simulink model "model"  (R2014a)
settings: Solver=VariableStepAuto  StartTime=0.0  StopTime=10.0  RelTol=1e-3
libraries: powerlib x113
settings Model: Creator=lej  LastModifiedBy=leimhofe
settings DataIOCC: SaveFormat=Dataset
settings OptimizationCC: SimCompilerOptimization=off
settings DebuggingCC: MergeDetectMultiDrivingBlocksExec=error  SolverPrmCheckMsg=none  FrameProcessingCompatibilityMsg=error  AllowSymbolicDim=off
settings HardwareCC: ProdBitPerPointer=64  ProdLargestAtomicFloat=Float  ProdIntDivRoundTo=Zero  ProdEndianess=LittleEndian  ProdWordSize=64  ProdHWDeviceType=Intel->x86-64 (Windows64)
settings RTWCC: RTWCompilerOptimization=off
settings GRTTargetCC: GeneratePreprocessorConditionals=Use local settings
settings ConfigComp: CovMetricSettings=dw  CovHtmlReporting=on  CovSaveCumulativeToWorkspaceVar=on  CovSaveSingleToWorkspaceVar=on  CovExternalEMLEnable=off

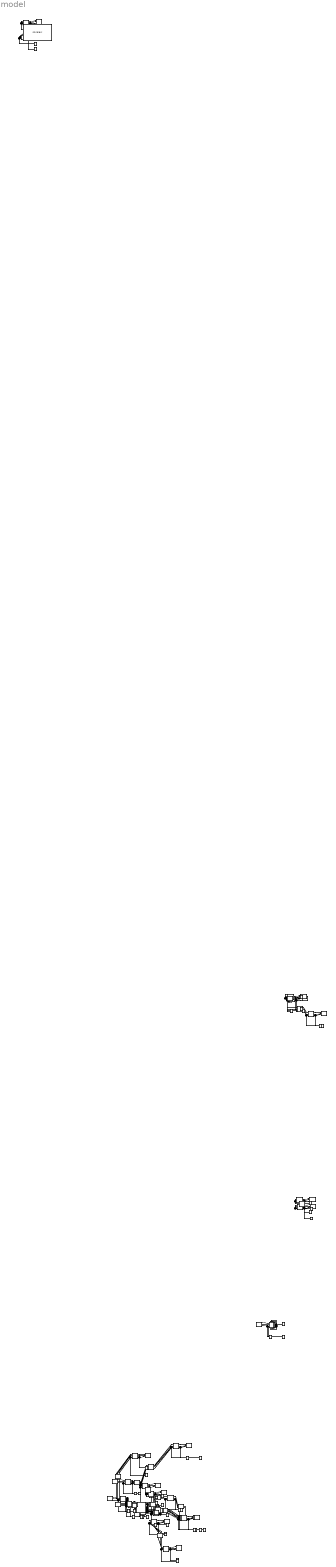
== system model ==
  note: 110000 Volts Power Line
  note: 220000 Volts Power Line
  note: 500000 Volts Power Line
  G_308292616_ : powerlib/Electrical Sources/Three-Phase Source  Voltage=220000  PhaseAngle=0  Frequency=60  InternalConnection=Yg  SpecifyImpedance=on  Resistance=0.8929  Inductance=16.58e-3  ShortCircuitLevel=100e6  BaseVoltage=220000  XRratio=7  BusType=swing  Pref=0  Qref=0  Qmin=-inf  Qmax=inf
  G_400202736_ : powerlib/Electrical Sources/Three-Phase Source  Voltage=220000  PhaseAngle=0  Frequency=60  InternalConnection=Yg  SpecifyImpedance=on  Resistance=0.8929  Inductance=16.58e-3  ShortCircuitLevel=100e6  BaseVoltage=220000  XRratio=7  BusType=swing  Pref=0  Qref=0  Qmin=-inf  Qmax=inf
  L_{251790836,251794098,277519190,306259034..306259035,306295540,306440155,308292630,315766015,318268202,400413519,400413521} (12 alike) : powerlib/Elements/Three-Phase Series RLC Load  LConnTagsString=A|B|C  Configuration=Y (grounded)  NominalVoltage=220000  NominalFrequency=60  ActivePower=100000  InductivePower=100  CapacitivePower=100  Measurements=None  LoadType=constant Z
  L_{272740093,306440153,315553115,401274166,401334056,401447890} (6 alike) : powerlib/Elements/Three-Phase Series RLC Load  LConnTagsString=A|B|C  Configuration=Y (grounded)  NominalVoltage=500000  NominalFrequency=60  ActivePower=100000  InductivePower=100  CapacitivePower=100  Measurements=None  LoadType=constant Z
  L_{306295536,307638314,317106134..317106135} (4 alike) : powerlib/Elements/Three-Phase Series RLC Load  LConnTagsString=A|B|C  Configuration=Y (grounded)  NominalVoltage=110000  NominalFrequency=60  ActivePower=100000  InductivePower=100  CapacitivePower=100  Measurements=None  LoadType=constant Z
  T_251790836__ : powerlib/Elements/Three-Phase Transformer (Two Windings)  Winding1Connection=Yg  UNITS=pu  NominalPower=[ 250e6 , 60 ]  Winding1=[220000,0.002,0.08]  Winding2Connection=Yg  Winding2=[220000,0.002,0.08]  SetSaturation=off  Rm=500  Lm=500  Saturation=[ 0,0 ; 0.0024,1.2 ; 1.0,1.52 ]  Hysteresis=off  DataFile='hysteresis'  SetInitialFlux=off  InitialFluxes=[ 0.8 , -0.8 , 0.7 ]  Measurements=None  MoreParameters=off  BreakLoop=off  DataType=off  TransfoNumber=1
  T_251794098__ : powerlib/Elements/Three-Phase Transformer (Two Windings)  Winding1Connection=Yg  UNITS=pu  NominalPower=[ 250e6 , 60 ]  Winding1=[220000,0.002,0.08]  Winding2Connection=Yg  Winding2=[220000,0.002,0.08]  SetSaturation=off  Rm=500  Lm=500  Saturation=[ 0,0 ; 0.0024,1.2 ; 1.0,1.52 ]  Hysteresis=off  DataFile='hysteresis'  SetInitialFlux=off  InitialFluxes=[ 0.8 , -0.8 , 0.7 ]  Measurements=None  MoreParameters=off  BreakLoop=off  DataType=off  TransfoNumber=1
  T_272740093_500000_Trạm_500KV_Phú_Mỹ : powerlib/Elements/Three-Phase Transformer (Two Windings)  Winding1Connection=Yg  UNITS=pu  NominalPower=[ 250e6 , 60 ]  Winding1=[500000,0.002,0.08]  Winding2Connection=Yg  Winding2=[500000,0.002,0.08]  SetSaturation=off  Rm=500  Lm=500  Saturation=[ 0,0 ; 0.0024,1.2 ; 1.0,1.52 ]  Hysteresis=off  DataFile='hysteresis'  SetInitialFlux=off  InitialFluxes=[ 0.8 , -0.8 , 0.7 ]  Measurements=None  MoreParameters=off  BreakLoop=off  DataType=off  TransfoNumber=1
  T_277519190__ : powerlib/Elements/Three-Phase Transformer (Two Windings)  Winding1Connection=Yg  UNITS=pu  NominalPower=[ 250e6 , 60 ]  Winding1=[220000,0.002,0.08]  Winding2Connection=Yg  Winding2=[220000,0.002,0.08]  SetSaturation=off  Rm=500  Lm=500  Saturation=[ 0,0 ; 0.0024,1.2 ; 1.0,1.52 ]  Hysteresis=off  DataFile='hysteresis'  SetInitialFlux=off  InitialFluxes=[ 0.8 , -0.8 , 0.7 ]  Measurements=None  MoreParameters=off  BreakLoop=off  DataType=off  TransfoNumber=1
  T_306259034__ : powerlib/Elements/Three-Phase Transformer (Two Windings)  Winding1Connection=Yg  UNITS=pu  NominalPower=[ 250e6 , 60 ]  Winding1=[220000,0.002,0.08]  Winding2Connection=Yg  Winding2=[220000,0.002,0.08]  SetSaturation=off  Rm=500  Lm=500  Saturation=[ 0,0 ; 0.0024,1.2 ; 1.0,1.52 ]  Hysteresis=off  DataFile='hysteresis'  SetInitialFlux=off  InitialFluxes=[ 0.8 , -0.8 , 0.7 ]  Measurements=None  MoreParameters=off  BreakLoop=off  DataType=off  TransfoNumber=1
  T_306259035__ : powerlib/Elements/Three-Phase Transformer (Two Windings)  Winding1Connection=Yg  UNITS=pu  NominalPower=[ 250e6 , 60 ]  Winding1=[220000,0.002,0.08]  Winding2Connection=Yg  Winding2=[220000,0.002,0.08]  SetSaturation=off  Rm=500  Lm=500  Saturation=[ 0,0 ; 0.0024,1.2 ; 1.0,1.52 ]  Hysteresis=off  DataFile='hysteresis'  SetInitialFlux=off  InitialFluxes=[ 0.8 , -0.8 , 0.7 ]  Measurements=None  MoreParameters=off  BreakLoop=off  DataType=off  TransfoNumber=1
  T_306295536_500000_Trạm_500KV_Nhà_Bè : powerlib/Elements/Three-Phase Transformer (Three Windings)  Winding1Connection=Yg  UNITS=pu  NominalPower=[ 250e6 , 60 ]  Winding1=[500000,0.002,0.08]  Winding2Connection=Yg  Winding2=[220000,0.002,0.08]  Winding3Connection=Yg  Winding3=[110000,0.002,0.08]  SetSaturation=off  Rm=500  Lm=500  Saturation=[ 0,0 ; 0.0024,1.2 ; 1.0,1.52 ]  Hysteresis=off  DataFile='hysteresis'  SetInitialFlux=off  InitialFluxes=[0.8 -0.8 0.7]  Measurements=None  MoreParameters=off  BreakLoop=off  DataType=off  TransfoNumber=1
  T_306295540__ : powerlib/Elements/Three-Phase Transformer (Two Windings)  Winding1Connection=Yg  UNITS=pu  NominalPower=[ 250e6 , 60 ]  Winding1=[220000,0.002,0.08]  Winding2Connection=Yg  Winding2=[220000,0.002,0.08]  SetSaturation=off  Rm=500  Lm=500  Saturation=[ 0,0 ; 0.0024,1.2 ; 1.0,1.52 ]  Hysteresis=off  DataFile='hysteresis'  SetInitialFlux=off  InitialFluxes=[ 0.8 , -0.8 , 0.7 ]  Measurements=None  MoreParameters=off  BreakLoop=off  DataType=off  TransfoNumber=1
  T_306440153__ : powerlib/Elements/Three-Phase Transformer (Two Windings)  Winding1Connection=Yg  UNITS=pu  NominalPower=[ 250e6 , 60 ]  Winding1=[500000,0.002,0.08]  Winding2Connection=Yg  Winding2=[500000,0.002,0.08]  SetSaturation=off  Rm=500  Lm=500  Saturation=[ 0,0 ; 0.0024,1.2 ; 1.0,1.52 ]  Hysteresis=off  DataFile='hysteresis'  SetInitialFlux=off  InitialFluxes=[ 0.8 , -0.8 , 0.7 ]  Measurements=None  MoreParameters=off  BreakLoop=off  DataType=off  TransfoNumber=1
  T_306440155__ : powerlib/Elements/Three-Phase Transformer (Two Windings)  Winding1Connection=Yg  UNITS=pu  NominalPower=[ 250e6 , 60 ]  Winding1=[220000,0.002,0.08]  Winding2Connection=Yg  Winding2=[220000,0.002,0.08]  SetSaturation=off  Rm=500  Lm=500  Saturation=[ 0,0 ; 0.0024,1.2 ; 1.0,1.52 ]  Hysteresis=off  DataFile='hysteresis'  SetInitialFlux=off  InitialFluxes=[ 0.8 , -0.8 , 0.7 ]  Measurements=None  MoreParameters=off  BreakLoop=off  DataType=off  TransfoNumber=1
  T_307638314__ : powerlib/Elements/Three-Phase Transformer (Two Windings)  Winding1Connection=Yg  UNITS=pu  NominalPower=[ 250e6 , 60 ]  Winding1=[220000,0.002,0.08]  Winding2Connection=Yg  Winding2=[110000,0.002,0.08]  SetSaturation=off  Rm=500  Lm=500  Saturation=[ 0,0 ; 0.0024,1.2 ; 1.0,1.52 ]  Hysteresis=off  DataFile='hysteresis'  SetInitialFlux=off  InitialFluxes=[ 0.8 , -0.8 , 0.7 ]  Measurements=None  MoreParameters=off  BreakLoop=off  DataType=off  TransfoNumber=1
  T_308292630__ : powerlib/Elements/Three-Phase Transformer (Two Windings)  Winding1Connection=Yg  UNITS=pu  NominalPower=[ 250e6 , 60 ]  Winding1=[220000,0.002,0.08]  Winding2Connection=Yg  Winding2=[220000,0.002,0.08]  SetSaturation=off  Rm=500  Lm=500  Saturation=[ 0,0 ; 0.0024,1.2 ; 1.0,1.52 ]  Hysteresis=off  DataFile='hysteresis'  SetInitialFlux=off  InitialFluxes=[ 0.8 , -0.8 , 0.7 ]  Measurements=None  MoreParameters=off  BreakLoop=off  DataType=off  TransfoNumber=1
  T_315553115__Phú_Lâm : powerlib/Elements/Three-Phase Transformer (Two Windings)  Winding1Connection=Yg  UNITS=pu  NominalPower=[ 250e6 , 60 ]  Winding1=[500000,0.002,0.08]  Winding2Connection=Yg  Winding2=[500000,0.002,0.08]  SetSaturation=off  Rm=500  Lm=500  Saturation=[ 0,0 ; 0.0024,1.2 ; 1.0,1.52 ]  Hysteresis=off  DataFile='hysteresis'  SetInitialFlux=off  InitialFluxes=[ 0.8 , -0.8 , 0.7 ]  Measurements=None  MoreParameters=off  BreakLoop=off  DataType=off  TransfoNumber=1
  T_315766015__ : powerlib/Elements/Three-Phase Transformer (Two Windings)  Winding1Connection=Yg  UNITS=pu  NominalPower=[ 250e6 , 60 ]  Winding1=[220000,0.002,0.08]  Winding2Connection=Yg  Winding2=[220000,0.002,0.08]  SetSaturation=off  Rm=500  Lm=500  Saturation=[ 0,0 ; 0.0024,1.2 ; 1.0,1.52 ]  Hysteresis=off  DataFile='hysteresis'  SetInitialFlux=off  InitialFluxes=[ 0.8 , -0.8 , 0.7 ]  Measurements=None  MoreParameters=off  BreakLoop=off  DataType=off  TransfoNumber=1
  T_317106134__ : powerlib/Elements/Three-Phase Transformer (Two Windings)  Winding1Connection=Yg  UNITS=pu  NominalPower=[ 250e6 , 60 ]  Winding1=[110000,0.002,0.08]  Winding2Connection=Yg  Winding2=[110000,0.002,0.08]  SetSaturation=off  Rm=500  Lm=500  Saturation=[ 0,0 ; 0.0024,1.2 ; 1.0,1.52 ]  Hysteresis=off  DataFile='hysteresis'  SetInitialFlux=off  InitialFluxes=[ 0.8 , -0.8 , 0.7 ]  Measurements=None  MoreParameters=off  BreakLoop=off  DataType=off  TransfoNumber=1
  T_317106135__ : powerlib/Elements/Three-Phase Transformer (Two Windings)  Winding1Connection=Yg  UNITS=pu  NominalPower=[ 250e6 , 60 ]  Winding1=[110000,0.002,0.08]  Winding2Connection=Yg  Winding2=[110000,0.002,0.08]  SetSaturation=off  Rm=500  Lm=500  Saturation=[ 0,0 ; 0.0024,1.2 ; 1.0,1.52 ]  Hysteresis=off  DataFile='hysteresis'  SetInitialFlux=off  InitialFluxes=[ 0.8 , -0.8 , 0.7 ]  Measurements=None  MoreParameters=off  BreakLoop=off  DataType=off  TransfoNumber=1
  T_318268202__ : powerlib/Elements/Three-Phase Transformer (Two Windings)  Winding1Connection=Yg  UNITS=pu  NominalPower=[ 250e6 , 60 ]  Winding1=[220000,0.002,0.08]  Winding2Connection=Yg  Winding2=[220000,0.002,0.08]  SetSaturation=off  Rm=500  Lm=500  Saturation=[ 0,0 ; 0.0024,1.2 ; 1.0,1.52 ]  Hysteresis=off  DataFile='hysteresis'  SetInitialFlux=off  InitialFluxes=[ 0.8 , -0.8 , 0.7 ]  Measurements=None  MoreParameters=off  BreakLoop=off  DataType=off  TransfoNumber=1
  T_400413519__ : powerlib/Elements/Three-Phase Transformer (Two Windings)  Winding1Connection=Yg  UNITS=pu  NominalPower=[ 250e6 , 60 ]  Winding1=[220000,0.002,0.08]  Winding2Connection=Yg  Winding2=[220000,0.002,0.08]  SetSaturation=off  Rm=500  Lm=500  Saturation=[ 0,0 ; 0.0024,1.2 ; 1.0,1.52 ]  Hysteresis=off  DataFile='hysteresis'  SetInitialFlux=off  InitialFluxes=[ 0.8 , -0.8 , 0.7 ]  Measurements=None  MoreParameters=off  BreakLoop=off  DataType=off  TransfoNumber=1
  T_400413521__ : powerlib/Elements/Three-Phase Transformer (Two Windings)  Winding1Connection=Yg  UNITS=pu  NominalPower=[ 250e6 , 60 ]  Winding1=[220000,0.002,0.08]  Winding2Connection=Yg  Winding2=[220000,0.002,0.08]  SetSaturation=off  Rm=500  Lm=500  Saturation=[ 0,0 ; 0.0024,1.2 ; 1.0,1.52 ]  Hysteresis=off  DataFile='hysteresis'  SetInitialFlux=off  InitialFluxes=[ 0.8 , -0.8 , 0.7 ]  Measurements=None  MoreParameters=off  BreakLoop=off  DataType=off  TransfoNumber=1
  T_401274166__ : powerlib/Elements/Three-Phase Transformer (Two Windings)  Winding1Connection=Yg  UNITS=pu  NominalPower=[ 250e6 , 60 ]  Winding1=[500000,0.002,0.08]  Winding2Connection=Yg  Winding2=[500000,0.002,0.08]  SetSaturation=off  Rm=500  Lm=500  Saturation=[ 0,0 ; 0.0024,1.2 ; 1.0,1.52 ]  Hysteresis=off  DataFile='hysteresis'  SetInitialFlux=off  InitialFluxes=[ 0.8 , -0.8 , 0.7 ]  Measurements=None  MoreParameters=off  BreakLoop=off  DataType=off  TransfoNumber=1
  T_401334056__ : powerlib/Elements/Three-Phase Transformer (Two Windings)  Winding1Connection=Yg  UNITS=pu  NominalPower=[ 250e6 , 60 ]  Winding1=[500000,0.002,0.08]  Winding2Connection=Yg  Winding2=[500000,0.002,0.08]  SetSaturation=off  Rm=500  Lm=500  Saturation=[ 0,0 ; 0.0024,1.2 ; 1.0,1.52 ]  Hysteresis=off  DataFile='hysteresis'  SetInitialFlux=off  InitialFluxes=[ 0.8 , -0.8 , 0.7 ]  Measurements=None  MoreParameters=off  BreakLoop=off  DataType=off  TransfoNumber=1
  T_401447890__ : powerlib/Elements/Three-Phase Transformer (Two Windings)  Winding1Connection=Yg  UNITS=pu  NominalPower=[ 250e6 , 60 ]  Winding1=[500000,0.002,0.08]  Winding2Connection=Yg  Winding2=[500000,0.002,0.08]  SetSaturation=off  Rm=500  Lm=500  Saturation=[ 0,0 ; 0.0024,1.2 ; 1.0,1.52 ]  Hysteresis=off  DataFile='hysteresis'  SetInitialFlux=off  InitialFluxes=[ 0.8 , -0.8 , 0.7 ]  Measurements=None  MoreParameters=off  BreakLoop=off  DataType=off  TransfoNumber=1
  _CN_251794098_220000_CN_251790836_220000 : powerlib/Elements/Distributed Parameters Line  Phases=3  Frequency=60  Resistance=[0.01273 0.3864]  Inductance="[0.9337e-3  4.1264e-3]"  Capacitance=[12.74e-9 7.751e-9]  Length=16.0988  x1=[0 0 0 0; 0.0001244 0 0 0; 0.0002488 0 0 0; 0.0003733 0 0 0; 0.0004977 0 0 0; 0.0006221 0 0 0]  x2=[0 0 0 0; 0.0001244 0 0 0; 0.0002488 0 0 0; 0.0003733 0 0 0; 0.0004977 0 0 0; 0.0006221 0 0 0]  x3=[0 0 0 0; 0.0001244 0 0 0; 0.0002488 0 0 0; 0.0003733 0 0 0; 0.0004977 0 0 0; 0.0006221 0 0 0]  x4=[0 0 0 0; 0.0001244 0 0 0; 0.0002488 0 0 0; 0.0003733 0 0 0; 0.0004977 0 0 0; 0.0006221 0 0 0]  x5=0  V1=ones(3,3)  V2=ones(3,3)  I1=ones(3,3)  I2=ones(3,3)  nHarmo=1  Measurements=None
  _CN_277519190_220000_CN_315766015_220000 : powerlib/Elements/Distributed Parameters Line  Phases=3  Frequency=60  Resistance=[0.01273 0.3864]  Inductance="[0.9337e-3  4.1264e-3]"  Capacitance=[12.74e-9 7.751e-9]  Length=24.7895  x1=[0 0 0 0; 0.0001244 0 0 0; 0.0002488 0 0 0; 0.0003733 0 0 0; 0.0004977 0 0 0; 0.0006221 0 0 0]  x2=[0 0 0 0; 0.0001244 0 0 0; 0.0002488 0 0 0; 0.0003733 0 0 0; 0.0004977 0 0 0; 0.0006221 0 0 0]  x3=[0 0 0 0; 0.0001244 0 0 0; 0.0002488 0 0 0; 0.0003733 0 0 0; 0.0004977 0 0 0; 0.0006221 0 0 0]  x4=[0 0 0 0; 0.0001244 0 0 0; 0.0002488 0 0 0; 0.0003733 0 0 0; 0.0004977 0 0 0; 0.0006221 0 0 0]  x5=0  V1=ones(3,3)  V2=ones(3,3)  I1=ones(3,3)  I2=ones(3,3)  nHarmo=1  Measurements=None
  _CN_306259035_220000_CN_306259034_220000 : powerlib/Elements/Distributed Parameters Line  Phases=3  Frequency=60  Resistance=[0.01273 0.3864]  Inductance="[0.9337e-3  4.1264e-3]"  Capacitance=[12.74e-9 7.751e-9]  Length=8.7616  x1=[0 0 0 0; 0.0001244 0 0 0; 0.0002488 0 0 0; 0.0003733 0 0 0; 0.0004977 0 0 0; 0.0006221 0 0 0]  x2=[0 0 0 0; 0.0001244 0 0 0; 0.0002488 0 0 0; 0.0003733 0 0 0; 0.0004977 0 0 0; 0.0006221 0 0 0]  x3=[0 0 0 0; 0.0001244 0 0 0; 0.0002488 0 0 0; 0.0003733 0 0 0; 0.0004977 0 0 0; 0.0006221 0 0 0]  x4=[0 0 0 0; 0.0001244 0 0 0; 0.0002488 0 0 0; 0.0003733 0 0 0; 0.0004977 0 0 0; 0.0006221 0 0 0]  x5=0  V1=ones(3,3)  V2=ones(3,3)  I1=ones(3,3)  I2=ones(3,3)  nHarmo=1  Measurements=None
  _CN_306259035_220000_CN_306440155_220000 : powerlib/Elements/Distributed Parameters Line  Phases=3  Frequency=60  Resistance=[0.01273 0.3864]  Inductance="[0.9337e-3  4.1264e-3]"  Capacitance=[12.74e-9 7.751e-9]  Length=62.0615  x1=[0 0 0 0; 0.0001244 0 0 0; 0.0002488 0 0 0; 0.0003733 0 0 0; 0.0004977 0 0 0; 0.0006221 0 0 0]  x2=[0 0 0 0; 0.0001244 0 0 0; 0.0002488 0 0 0; 0.0003733 0 0 0; 0.0004977 0 0 0; 0.0006221 0 0 0]  x3=[0 0 0 0; 0.0001244 0 0 0; 0.0002488 0 0 0; 0.0003733 0 0 0; 0.0004977 0 0 0; 0.0006221 0 0 0]  x4=[0 0 0 0; 0.0001244 0 0 0; 0.0002488 0 0 0; 0.0003733 0 0 0; 0.0004977 0 0 0; 0.0006221 0 0 0]  x5=0  V1=ones(3,3)  V2=ones(3,3)  I1=ones(3,3)  I2=ones(3,3)  nHarmo=1  Measurements=None
  _CN_306259035_220000_CN_318268202_220000 : powerlib/Elements/Distributed Parameters Line  Phases=3  Frequency=60  Resistance=[0.01273 0.3864]  Inductance="[0.9337e-3  4.1264e-3]"  Capacitance=[12.74e-9 7.751e-9]  Length=14.6107  x1=[0 0 0 0; 0.0001244 0 0 0; 0.0002488 0 0 0; 0.0003733 0 0 0; 0.0004977 0 0 0; 0.0006221 0 0 0]  x2=[0 0 0 0; 0.0001244 0 0 0; 0.0002488 0 0 0; 0.0003733 0 0 0; 0.0004977 0 0 0; 0.0006221 0 0 0]  x3=[0 0 0 0; 0.0001244 0 0 0; 0.0002488 0 0 0; 0.0003733 0 0 0; 0.0004977 0 0 0; 0.0006221 0 0 0]  x4=[0 0 0 0; 0.0001244 0 0 0; 0.0002488 0 0 0; 0.0003733 0 0 0; 0.0004977 0 0 0; 0.0006221 0 0 0]  x5=0  V1=ones(3,3)  V2=ones(3,3)  I1=ones(3,3)  I2=ones(3,3)  nHarmo=1  Measurements=None
  _CN_306295536_500000_CN_272740093_500000 : powerlib/Elements/Distributed Parameters Line  Phases=3  Frequency=60  Resistance=[0.01273 0.3864]  Inductance="[0.9337e-3  4.1264e-3]"  Capacitance=[12.74e-9 7.751e-9]  Length=42.5301  x1=[0 0 0 0; 0.0001244 0 0 0; 0.0002488 0 0 0; 0.0003733 0 0 0; 0.0004977 0 0 0; 0.0006221 0 0 0]  x2=[0 0 0 0; 0.0001244 0 0 0; 0.0002488 0 0 0; 0.0003733 0 0 0; 0.0004977 0 0 0; 0.0006221 0 0 0]  x3=[0 0 0 0; 0.0001244 0 0 0; 0.0002488 0 0 0; 0.0003733 0 0 0; 0.0004977 0 0 0; 0.0006221 0 0 0]  x4=[0 0 0 0; 0.0001244 0 0 0; 0.0002488 0 0 0; 0.0003733 0 0 0; 0.0004977 0 0 0; 0.0006221 0 0 0]  x5=0  V1=ones(3,3)  V2=ones(3,3)  I1=ones(3,3)  I2=ones(3,3)  nHarmo=1  Measurements=None
  _CN_306295536_500000_CN_315553115_500000 : powerlib/Elements/Distributed Parameters Line  Phases=3  Frequency=60  Resistance=[0.01273 0.3864]  Inductance="[0.9337e-3  4.1264e-3]"  Capacitance=[12.74e-9 7.751e-9]  Length=16.513  x1=[0 0 0 0; 0.0001244 0 0 0; 0.0002488 0 0 0; 0.0003733 0 0 0; 0.0004977 0 0 0; 0.0006221 0 0 0]  x2=[0 0 0 0; 0.0001244 0 0 0; 0.0002488 0 0 0; 0.0003733 0 0 0; 0.0004977 0 0 0; 0.0006221 0 0 0]  x3=[0 0 0 0; 0.0001244 0 0 0; 0.0002488 0 0 0; 0.0003733 0 0 0; 0.0004977 0 0 0; 0.0006221 0 0 0]  x4=[0 0 0 0; 0.0001244 0 0 0; 0.0002488 0 0 0; 0.0003733 0 0 0; 0.0004977 0 0 0; 0.0006221 0 0 0]  x5=0  V1=ones(3,3)  V2=ones(3,3)  I1=ones(3,3)  I2=ones(3,3)  nHarmo=1  Measurements=None
  _CN_306295540_220000_CN_277519190_220000 : powerlib/Elements/Distributed Parameters Line  Phases=3  Frequency=60  Resistance=[0.01273 0.3864]  Inductance="[0.9337e-3  4.1264e-3]"  Capacitance=[12.74e-9 7.751e-9]  Length=37.7221  x1=[0 0 0 0; 0.0001244 0 0 0; 0.0002488 0 0 0; 0.0003733 0 0 0; 0.0004977 0 0 0; 0.0006221 0 0 0]  x2=[0 0 0 0; 0.0001244 0 0 0; 0.0002488 0 0 0; 0.0003733 0 0 0; 0.0004977 0 0 0; 0.0006221 0 0 0]  x3=[0 0 0 0; 0.0001244 0 0 0; 0.0002488 0 0 0; 0.0003733 0 0 0; 0.0004977 0 0 0; 0.0006221 0 0 0]  x4=[0 0 0 0; 0.0001244 0 0 0; 0.0002488 0 0 0; 0.0003733 0 0 0; 0.0004977 0 0 0; 0.0006221 0 0 0]  x5=0  V1=ones(3,3)  V2=ones(3,3)  I1=ones(3,3)  I2=ones(3,3)  nHarmo=1  Measurements=None
  _CN_306295540_220000_CN_306259034_220000 : powerlib/Elements/Distributed Parameters Line  Phases=3  Frequency=60  Resistance=[0.01273 0.3864]  Inductance="[0.9337e-3  4.1264e-3]"  Capacitance=[12.74e-9 7.751e-9]  Length=20.2471  x1=[0 0 0 0; 0.0001244 0 0 0; 0.0002488 0 0 0; 0.0003733 0 0 0; 0.0004977 0 0 0; 0.0006221 0 0 0]  x2=[0 0 0 0; 0.0001244 0 0 0; 0.0002488 0 0 0; 0.0003733 0 0 0; 0.0004977 0 0 0; 0.0006221 0 0 0]  x3=[0 0 0 0; 0.0001244 0 0 0; 0.0002488 0 0 0; 0.0003733 0 0 0; 0.0004977 0 0 0; 0.0006221 0 0 0]  x4=[0 0 0 0; 0.0001244 0 0 0; 0.0002488 0 0 0; 0.0003733 0 0 0; 0.0004977 0 0 0; 0.0006221 0 0 0]  x5=0  V1=ones(3,3)  V2=ones(3,3)  I1=ones(3,3)  I2=ones(3,3)  nHarmo=1  Measurements=None
  _CN_306295540_220000_CN_306295536_220000 : powerlib/Elements/Distributed Parameters Line  Phases=3  Frequency=60  Resistance=[0.01273 0.3864]  Inductance="[0.9337e-3  4.1264e-3]"  Capacitance=[12.74e-9 7.751e-9]  Length=63.1316  x1=[0 0 0 0; 0.0001244 0 0 0; 0.0002488 0 0 0; 0.0003733 0 0 0; 0.0004977 0 0 0; 0.0006221 0 0 0]  x2=[0 0 0 0; 0.0001244 0 0 0; 0.0002488 0 0 0; 0.0003733 0 0 0; 0.0004977 0 0 0; 0.0006221 0 0 0]  x3=[0 0 0 0; 0.0001244 0 0 0; 0.0002488 0 0 0; 0.0003733 0 0 0; 0.0004977 0 0 0; 0.0006221 0 0 0]  x4=[0 0 0 0; 0.0001244 0 0 0; 0.0002488 0 0 0; 0.0003733 0 0 0; 0.0004977 0 0 0; 0.0006221 0 0 0]  x5=0  V1=ones(3,3)  V2=ones(3,3)  I1=ones(3,3)  I2=ones(3,3)  nHarmo=1  Measurements=None
  _CN_306295540_220000_CN_400202736_220000 : powerlib/Elements/Distributed Parameters Line  Phases=3  Frequency=60  Resistance=[0.01273 0.3864]  Inductance="[0.9337e-3  4.1264e-3]"  Capacitance=[12.74e-9 7.751e-9]  Length=0.74989  x1=[0 0 0 0; 0.0001244 0 0 0; 0.0002488 0 0 0; 0.0003733 0 0 0; 0.0004977 0 0 0; 0.0006221 0 0 0]  x2=[0 0 0 0; 0.0001244 0 0 0; 0.0002488 0 0 0; 0.0003733 0 0 0; 0.0004977 0 0 0; 0.0006221 0 0 0]  x3=[0 0 0 0; 0.0001244 0 0 0; 0.0002488 0 0 0; 0.0003733 0 0 0; 0.0004977 0 0 0; 0.0006221 0 0 0]  x4=[0 0 0 0; 0.0001244 0 0 0; 0.0002488 0 0 0; 0.0003733 0 0 0; 0.0004977 0 0 0; 0.0006221 0 0 0]  x5=0  V1=ones(3,3)  V2=ones(3,3)  I1=ones(3,3)  I2=ones(3,3)  nHarmo=1  Measurements=None
  _CN_306440153_500000_CN_315553115_500000 : powerlib/Elements/Distributed Parameters Line  Phases=3  Frequency=60  Resistance=[0.01273 0.3864]  Inductance="[0.9337e-3  4.1264e-3]"  Capacitance=[12.74e-9 7.751e-9]  Length=49.1318  x1=[0 0 0 0; 0.0001244 0 0 0; 0.0002488 0 0 0; 0.0003733 0 0 0; 0.0004977 0 0 0; 0.0006221 0 0 0]  x2=[0 0 0 0; 0.0001244 0 0 0; 0.0002488 0 0 0; 0.0003733 0 0 0; 0.0004977 0 0 0; 0.0006221 0 0 0]  x3=[0 0 0 0; 0.0001244 0 0 0; 0.0002488 0 0 0; 0.0003733 0 0 0; 0.0004977 0 0 0; 0.0006221 0 0 0]  x4=[0 0 0 0; 0.0001244 0 0 0; 0.0002488 0 0 0; 0.0003733 0 0 0; 0.0004977 0 0 0; 0.0006221 0 0 0]  x5=0  V1=ones(3,3)  V2=ones(3,3)  I1=ones(3,3)  I2=ones(3,3)  nHarmo=1  Measurements=None
  _CN_307638314_110000_CN_306295536_110000 : powerlib/Elements/Distributed Parameters Line  Phases=3  Frequency=60  Resistance=[0.01273 0.3864]  Inductance="[0.9337e-3  4.1264e-3]"  Capacitance=[12.74e-9 7.751e-9]  Length=6.8086  x1=[0 0 0 0; 0.0001244 0 0 0; 0.0002488 0 0 0; 0.0003733 0 0 0; 0.0004977 0 0 0; 0.0006221 0 0 0]  x2=[0 0 0 0; 0.0001244 0 0 0; 0.0002488 0 0 0; 0.0003733 0 0 0; 0.0004977 0 0 0; 0.0006221 0 0 0]  x3=[0 0 0 0; 0.0001244 0 0 0; 0.0002488 0 0 0; 0.0003733 0 0 0; 0.0004977 0 0 0; 0.0006221 0 0 0]  x4=[0 0 0 0; 0.0001244 0 0 0; 0.0002488 0 0 0; 0.0003733 0 0 0; 0.0004977 0 0 0; 0.0006221 0 0 0]  x5=0  V1=ones(3,3)  V2=ones(3,3)  I1=ones(3,3)  I2=ones(3,3)  nHarmo=1  Measurements=None
  _CN_307638314_220000_CN_306295536_220000 : powerlib/Elements/Distributed Parameters Line  Phases=3  Frequency=60  Resistance=[0.01273 0.3864]  Inductance="[0.9337e-3  4.1264e-3]"  Capacitance=[12.74e-9 7.751e-9]  Length=6.5587  x1=[0 0 0 0; 0.0001244 0 0 0; 0.0002488 0 0 0; 0.0003733 0 0 0; 0.0004977 0 0 0; 0.0006221 0 0 0]  x2=[0 0 0 0; 0.0001244 0 0 0; 0.0002488 0 0 0; 0.0003733 0 0 0; 0.0004977 0 0 0; 0.0006221 0 0 0]  x3=[0 0 0 0; 0.0001244 0 0 0; 0.0002488 0 0 0; 0.0003733 0 0 0; 0.0004977 0 0 0; 0.0006221 0 0 0]  x4=[0 0 0 0; 0.0001244 0 0 0; 0.0002488 0 0 0; 0.0003733 0 0 0; 0.0004977 0 0 0; 0.0006221 0 0 0]  x5=0  V1=ones(3,3)  V2=ones(3,3)  I1=ones(3,3)  I2=ones(3,3)  nHarmo=1  Measurements=None
  _CN_308292630_220000_CN_308292616_220000 : powerlib/Elements/Distributed Parameters Line  Phases=3  Frequency=60  Resistance=[0.01273 0.3864]  Inductance="[0.9337e-3  4.1264e-3]"  Capacitance=[12.74e-9 7.751e-9]  Length=0.39244  x1=[0 0 0 0; 0.0001244 0 0 0; 0.0002488 0 0 0; 0.0003733 0 0 0; 0.0004977 0 0 0; 0.0006221 0 0 0]  x2=[0 0 0 0; 0.0001244 0 0 0; 0.0002488 0 0 0; 0.0003733 0 0 0; 0.0004977 0 0 0; 0.0006221 0 0 0]  x3=[0 0 0 0; 0.0001244 0 0 0; 0.0002488 0 0 0; 0.0003733 0 0 0; 0.0004977 0 0 0; 0.0006221 0 0 0]  x4=[0 0 0 0; 0.0001244 0 0 0; 0.0002488 0 0 0; 0.0003733 0 0 0; 0.0004977 0 0 0; 0.0006221 0 0 0]  x5=0  V1=ones(3,3)  V2=ones(3,3)  I1=ones(3,3)  I2=ones(3,3)  nHarmo=1  Measurements=None
  _CN_317106134_110000_CN_317106135_110000 : powerlib/Elements/Distributed Parameters Line  Phases=3  Frequency=60  Resistance=[0.01273 0.3864]  Inductance="[0.9337e-3  4.1264e-3]"  Capacitance=[12.74e-9 7.751e-9]  Length=23.915  x1=[0 0 0 0; 0.0001244 0 0 0; 0.0002488 0 0 0; 0.0003733 0 0 0; 0.0004977 0 0 0; 0.0006221 0 0 0]  x2=[0 0 0 0; 0.0001244 0 0 0; 0.0002488 0 0 0; 0.0003733 0 0 0; 0.0004977 0 0 0; 0.0006221 0 0 0]  x3=[0 0 0 0; 0.0001244 0 0 0; 0.0002488 0 0 0; 0.0003733 0 0 0; 0.0004977 0 0 0; 0.0006221 0 0 0]  x4=[0 0 0 0; 0.0001244 0 0 0; 0.0002488 0 0 0; 0.0003733 0 0 0; 0.0004977 0 0 0; 0.0006221 0 0 0]  x5=0  V1=ones(3,3)  V2=ones(3,3)  I1=ones(3,3)  I2=ones(3,3)  nHarmo=1  Measurements=None
  _CN_400413519_220000_CN_400413521_220000 : powerlib/Elements/Distributed Parameters Line  Phases=3  Frequency=60  Resistance=[0.01273 0.3864]  Inductance="[0.9337e-3  4.1264e-3]"  Capacitance=[12.74e-9 7.751e-9]  Length=10.5428  x1=[0 0 0 0; 0.0001244 0 0 0; 0.0002488 0 0 0; 0.0003733 0 0 0; 0.0004977 0 0 0; 0.0006221 0 0 0]  x2=[0 0 0 0; 0.0001244 0 0 0; 0.0002488 0 0 0; 0.0003733 0 0 0; 0.0004977 0 0 0; 0.0006221 0 0 0]  x3=[0 0 0 0; 0.0001244 0 0 0; 0.0002488 0 0 0; 0.0003733 0 0 0; 0.0004977 0 0 0; 0.0006221 0 0 0]  x4=[0 0 0 0; 0.0001244 0 0 0; 0.0002488 0 0 0; 0.0003733 0 0 0; 0.0004977 0 0 0; 0.0006221 0 0 0]  x5=0  V1=ones(3,3)  V2=ones(3,3)  I1=ones(3,3)  I2=ones(3,3)  nHarmo=1  Measurements=None
  _CN_401334056_500000_CN_401274166_500000 : powerlib/Elements/Distributed Parameters Line  Phases=3  Frequency=60  Resistance=[0.01273 0.3864]  Inductance="[0.9337e-3  4.1264e-3]"  Capacitance=[12.74e-9 7.751e-9]  Length=20.0223  x1=[0 0 0 0; 0.0001244 0 0 0; 0.0002488 0 0 0; 0.0003733 0 0 0; 0.0004977 0 0 0; 0.0006221 0 0 0]  x2=[0 0 0 0; 0.0001244 0 0 0; 0.0002488 0 0 0; 0.0003733 0 0 0; 0.0004977 0 0 0; 0.0006221 0 0 0]  x3=[0 0 0 0; 0.0001244 0 0 0; 0.0002488 0 0 0; 0.0003733 0 0 0; 0.0004977 0 0 0; 0.0006221 0 0 0]  x4=[0 0 0 0; 0.0001244 0 0 0; 0.0002488 0 0 0; 0.0003733 0 0 0; 0.0004977 0 0 0; 0.0006221 0 0 0]  x5=0  V1=ones(3,3)  V2=ones(3,3)  I1=ones(3,3)  I2=ones(3,3)  nHarmo=1  Measurements=None
  _CN_401334056_500000_CN_401447890_500000 : powerlib/Elements/Distributed Parameters Line  Phases=3  Frequency=60  Resistance=[0.01273 0.3864]  Inductance="[0.9337e-3  4.1264e-3]"  Capacitance=[12.74e-9 7.751e-9]  Length=2.1964  x1=[0 0 0 0; 0.0001244 0 0 0; 0.0002488 0 0 0; 0.0003733 0 0 0; 0.0004977 0 0 0; 0.0006221 0 0 0]  x2=[0 0 0 0; 0.0001244 0 0 0; 0.0002488 0 0 0; 0.0003733 0 0 0; 0.0004977 0 0 0; 0.0006221 0 0 0]  x3=[0 0 0 0; 0.0001244 0 0 0; 0.0002488 0 0 0; 0.0003733 0 0 0; 0.0004977 0 0 0; 0.0006221 0 0 0]  x4=[0 0 0 0; 0.0001244 0 0 0; 0.0002488 0 0 0; 0.0003733 0 0 0; 0.0004977 0 0 0; 0.0006221 0 0 0]  x5=0  V1=ones(3,3)  V2=ones(3,3)  I1=ones(3,3)  I2=ones(3,3)  nHarmo=1  Measurements=None
  bus1 : powerlib/Measurements/Load Flow Bus  LConnTagsString=a  ID=bus1  Vbase=110000  Vref=1  Vangle=0  VLF=1  angleLF=0
      settings: AttributesFormatString=|
      | %<ID>
      | %<Vbase>V
      | %<VLF>pu
      | %<angleLF>deg.
      | %<Name>
  bus10 : powerlib/Measurements/Load Flow Bus  LConnTagsString=a  ID=bus10  Vbase=220000  Vref=1  Vangle=0  VLF=1  angleLF=0
      settings: AttributesFormatString=|
      | %<ID>
      | %<Vbase>V
      | %<VLF>pu
      | %<angleLF>deg.
      | %<Name>
  bus11 : powerlib/Measurements/Load Flow Bus  LConnTagsString=a  ID=bus11  Vbase=220000  Vref=1  Vangle=0  VLF=1  angleLF=0
      settings: AttributesFormatString=|
      | %<ID>
      | %<Vbase>V
      | %<VLF>pu
      | %<angleLF>deg.
      | %<Name>
  bus12 : powerlib/Measurements/Load Flow Bus  LConnTagsString=a  ID=bus12  Vbase=220000  Vref=1  Vangle=0  VLF=1  angleLF=0
      settings: AttributesFormatString=|
      | %<ID>
      | %<Vbase>V
      | %<VLF>pu
      | %<angleLF>deg.
      | %<Name>
  bus13 : powerlib/Measurements/Load Flow Bus  LConnTagsString=a  ID=bus13  Vbase=220000  Vref=1  Vangle=0  VLF=1  angleLF=0
      settings: AttributesFormatString=|
      | %<ID>
      | %<Vbase>V
      | %<VLF>pu
      | %<angleLF>deg.
      | %<Name>
  bus14 : powerlib/Measurements/Load Flow Bus  LConnTagsString=a  ID=bus14  Vbase=220000  Vref=1  Vangle=0  VLF=1  angleLF=0
      settings: AttributesFormatString=|
      | %<ID>
      | %<Vbase>V
      | %<VLF>pu
      | %<angleLF>deg.
      | %<Name>
  bus15 : powerlib/Measurements/Load Flow Bus  LConnTagsString=a  ID=bus15  Vbase=220000  Vref=1  Vangle=0  VLF=1  angleLF=0
      settings: AttributesFormatString=|
      | %<ID>
      | %<Vbase>V
      | %<VLF>pu
      | %<angleLF>deg.
      | %<Name>
  bus16 : powerlib/Measurements/Load Flow Bus  LConnTagsString=a  ID=bus16  Vbase=220000  Vref=1  Vangle=0  VLF=1  angleLF=0
      settings: AttributesFormatString=|
      | %<ID>
      | %<Vbase>V
      | %<VLF>pu
      | %<angleLF>deg.
      | %<Name>
  bus17 : powerlib/Measurements/Load Flow Bus  LConnTagsString=a  ID=bus17  Vbase=220000  Vref=1  Vangle=0  VLF=1  angleLF=0
      settings: AttributesFormatString=|
      | %<ID>
      | %<Vbase>V
      | %<VLF>pu
      | %<angleLF>deg.
      | %<Name>
  bus18 : powerlib/Measurements/Load Flow Bus  LConnTagsString=a  ID=bus18  Vbase=220000  Vref=1  Vangle=0  VLF=1  angleLF=0
      settings: AttributesFormatString=|
      | %<ID>
      | %<Vbase>V
      | %<VLF>pu
      | %<angleLF>deg.
      | %<Name>
  bus19 : powerlib/Measurements/Load Flow Bus  LConnTagsString=a  ID=bus19  Vbase=220000  Vref=1  Vangle=0  VLF=1  angleLF=0
      settings: AttributesFormatString=|
      | %<ID>
      | %<Vbase>V
      | %<VLF>pu
      | %<angleLF>deg.
      | %<Name>
  bus2 : powerlib/Measurements/Load Flow Bus  LConnTagsString=a  ID=bus2  Vbase=110000  Vref=1  Vangle=0  VLF=1  angleLF=0
      settings: AttributesFormatString=|
      | %<ID>
      | %<Vbase>V
      | %<VLF>pu
      | %<angleLF>deg.
      | %<Name>
  bus20 : powerlib/Measurements/Load Flow Bus  LConnTagsString=a  ID=bus20  Vbase=220000  Vref=1  Vangle=0  VLF=1  angleLF=0
      settings: AttributesFormatString=|
      | %<ID>
      | %<Vbase>V
      | %<VLF>pu
      | %<angleLF>deg.
      | %<Name>
  bus21 : powerlib/Measurements/Load Flow Bus  LConnTagsString=a  ID=bus21  Vbase=500000  Vref=1  Vangle=0  VLF=1  angleLF=0
      settings: AttributesFormatString=|
      | %<ID>
      | %<Vbase>V
      | %<VLF>pu
      | %<angleLF>deg.
      | %<Name>
  bus22 : powerlib/Measurements/Load Flow Bus  LConnTagsString=a  ID=bus22  Vbase=500000  Vref=1  Vangle=0  VLF=1  angleLF=0
      settings: AttributesFormatString=|
      | %<ID>
      | %<Vbase>V
      | %<VLF>pu
      | %<angleLF>deg.
      | %<Name>
  bus23 : powerlib/Measurements/Load Flow Bus  LConnTagsString=a  ID=bus23  Vbase=500000  Vref=1  Vangle=0  VLF=1  angleLF=0
      settings: AttributesFormatString=|
      | %<ID>
      | %<Vbase>V
      | %<VLF>pu
      | %<angleLF>deg.
      | %<Name>
  bus24 : powerlib/Measurements/Load Flow Bus  LConnTagsString=a  ID=bus24  Vbase=500000  Vref=1  Vangle=0  VLF=1  angleLF=0
      settings: AttributesFormatString=|
      | %<ID>
      | %<Vbase>V
      | %<VLF>pu
      | %<angleLF>deg.
      | %<Name>
  bus25 : powerlib/Measurements/Load Flow Bus  LConnTagsString=a  ID=bus25  Vbase=500000  Vref=1  Vangle=0  VLF=1  angleLF=0
      settings: AttributesFormatString=|
      | %<ID>
      | %<Vbase>V
      | %<VLF>pu
      | %<angleLF>deg.
      | %<Name>
  bus26 : powerlib/Measurements/Load Flow Bus  LConnTagsString=a  ID=bus26  Vbase=500000  Vref=1  Vangle=0  VLF=1  angleLF=0
      settings: AttributesFormatString=|
      | %<ID>
      | %<Vbase>V
      | %<VLF>pu
      | %<angleLF>deg.
      | %<Name>
  bus27 : powerlib/Measurements/Load Flow Bus  LConnTagsString=a  ID=bus27  Vbase=500000  Vref=1  Vangle=0  VLF=1  angleLF=0
      settings: AttributesFormatString=|
      | %<ID>
      | %<Vbase>V
      | %<VLF>pu
      | %<angleLF>deg.
      | %<Name>
  bus28 : powerlib/Measurements/Load Flow Bus  LConnTagsString=a  ID=bus28  Vbase=110000  Vref=1  Vangle=0  VLF=1  angleLF=0
      settings: AttributesFormatString=|
      | %<ID>
      | %<Vbase>V
      | %<VLF>pu
      | %<angleLF>deg.
      | %<Name>
  bus29 : powerlib/Measurements/Load Flow Bus  LConnTagsString=a  ID=bus29  Vbase=110000  Vref=1  Vangle=0  VLF=1  angleLF=0
      settings: AttributesFormatString=|
      | %<ID>
      | %<Vbase>V
      | %<VLF>pu
      | %<angleLF>deg.
      | %<Name>
  bus3 : powerlib/Measurements/Load Flow Bus  LConnTagsString=a  ID=bus3  Vbase=110000  Vref=1  Vangle=0  VLF=1  angleLF=0
      settings: AttributesFormatString=|
      | %<ID>
      | %<Vbase>V
      | %<VLF>pu
      | %<angleLF>deg.
      | %<Name>
  bus30 : powerlib/Measurements/Load Flow Bus  LConnTagsString=a  ID=bus30  Vbase=220000  Vref=1  Vangle=0  VLF=1  angleLF=0
      settings: AttributesFormatString=|
      | %<ID>
      | %<Vbase>V
      | %<VLF>pu
      | %<angleLF>deg.
      | %<Name>
  bus31 : powerlib/Measurements/Load Flow Bus  LConnTagsString=a  ID=bus31  Vbase=220000  Vref=1  Vangle=0  VLF=1  angleLF=0
      settings: AttributesFormatString=|
      | %<ID>
      | %<Vbase>V
      | %<VLF>pu
      | %<angleLF>deg.
      | %<Name>
  bus32 : powerlib/Measurements/Load Flow Bus  LConnTagsString=a  ID=bus32  Vbase=220000  Vref=1  Vangle=0  VLF=1  angleLF=0
      settings: AttributesFormatString=|
      | %<ID>
      | %<Vbase>V
      | %<VLF>pu
      | %<angleLF>deg.
      | %<Name>
  bus33 : powerlib/Measurements/Load Flow Bus  LConnTagsString=a  ID=bus33  Vbase=220000  Vref=1  Vangle=0  VLF=1  angleLF=0
      settings: AttributesFormatString=|
      | %<ID>
      | %<Vbase>V
      | %<VLF>pu
      | %<angleLF>deg.
      | %<Name>
  bus34 : powerlib/Measurements/Load Flow Bus  LConnTagsString=a  ID=bus34  Vbase=220000  Vref=1  Vangle=0  VLF=1  angleLF=0
      settings: AttributesFormatString=|
      | %<ID>
      | %<Vbase>V
      | %<VLF>pu
      | %<angleLF>deg.
      | %<Name>
  bus35 : powerlib/Measurements/Load Flow Bus  LConnTagsString=a  ID=bus35  Vbase=220000  Vref=1  Vangle=0  VLF=1  angleLF=0
      settings: AttributesFormatString=|
      | %<ID>
      | %<Vbase>V
      | %<VLF>pu
      | %<angleLF>deg.
      | %<Name>
  bus36 : powerlib/Measurements/Load Flow Bus  LConnTagsString=a  ID=bus36  Vbase=220000  Vref=1  Vangle=0  VLF=1  angleLF=0
      settings: AttributesFormatString=|
      | %<ID>
      | %<Vbase>V
      | %<VLF>pu
      | %<angleLF>deg.
      | %<Name>
  bus37 : powerlib/Measurements/Load Flow Bus  LConnTagsString=a  ID=bus37  Vbase=220000  Vref=1  Vangle=0  VLF=1  angleLF=0
      settings: AttributesFormatString=|
      | %<ID>
      | %<Vbase>V
      | %<VLF>pu
      | %<angleLF>deg.
      | %<Name>
  bus38 : powerlib/Measurements/Load Flow Bus  LConnTagsString=a  ID=bus38  Vbase=220000  Vref=1  Vangle=0  VLF=1  angleLF=0
      settings: AttributesFormatString=|
      | %<ID>
      | %<Vbase>V
      | %<VLF>pu
      | %<angleLF>deg.
      | %<Name>
  bus39 : powerlib/Measurements/Load Flow Bus  LConnTagsString=a  ID=bus39  Vbase=220000  Vref=1  Vangle=0  VLF=1  angleLF=0
      settings: AttributesFormatString=|
      | %<ID>
      | %<Vbase>V
      | %<VLF>pu
      | %<angleLF>deg.
      | %<Name>
  bus4 : powerlib/Measurements/Load Flow Bus  LConnTagsString=a  ID=bus4  Vbase=110000  Vref=1  Vangle=0  VLF=1  angleLF=0
      settings: AttributesFormatString=|
      | %<ID>
      | %<Vbase>V
      | %<VLF>pu
      | %<angleLF>deg.
      | %<Name>
  bus40 : powerlib/Measurements/Load Flow Bus  LConnTagsString=a  ID=bus40  Vbase=220000  Vref=1  Vangle=0  VLF=1  angleLF=0
      settings: AttributesFormatString=|
      | %<ID>
      | %<Vbase>V
      | %<VLF>pu
      | %<angleLF>deg.
      | %<Name>
  bus41 : powerlib/Measurements/Load Flow Bus  LConnTagsString=a  ID=bus41  Vbase=220000  Vref=1  Vangle=0  VLF=1  angleLF=0
      settings: AttributesFormatString=|
      | %<ID>
      | %<Vbase>V
      | %<VLF>pu
      | %<angleLF>deg.
      | %<Name>
  bus42 : powerlib/Measurements/Load Flow Bus  LConnTagsString=a  ID=bus42  Vbase=500000  Vref=1  Vangle=0  VLF=1  angleLF=0
      settings: AttributesFormatString=|
      | %<ID>
      | %<Vbase>V
      | %<VLF>pu
      | %<angleLF>deg.
      | %<Name>
  bus43 : powerlib/Measurements/Load Flow Bus  LConnTagsString=a  ID=bus43  Vbase=500000  Vref=1  Vangle=0  VLF=1  angleLF=0
      settings: AttributesFormatString=|
      | %<ID>
      | %<Vbase>V
      | %<VLF>pu
      | %<angleLF>deg.
      | %<Name>
  bus44 : powerlib/Measurements/Load Flow Bus  LConnTagsString=a  ID=bus44  Vbase=500000  Vref=1  Vangle=0  VLF=1  angleLF=0
      settings: AttributesFormatString=|
      | %<ID>
      | %<Vbase>V
      | %<VLF>pu
      | %<angleLF>deg.
      | %<Name>
  bus45 : powerlib/Measurements/Load Flow Bus  LConnTagsString=a  ID=bus45  Vbase=500000  Vref=1  Vangle=0  VLF=1  angleLF=0
      settings: AttributesFormatString=|
      | %<ID>
      | %<Vbase>V
      | %<VLF>pu
      | %<angleLF>deg.
      | %<Name>
  bus46 : powerlib/Measurements/Load Flow Bus  LConnTagsString=a  ID=bus46  Vbase=500000  Vref=1  Vangle=0  VLF=1  angleLF=0
      settings: AttributesFormatString=|
      | %<ID>
      | %<Vbase>V
      | %<VLF>pu
      | %<angleLF>deg.
      | %<Name>
  bus47 : powerlib/Measurements/Load Flow Bus  LConnTagsString=a  ID=bus47  Vbase=500000  Vref=1  Vangle=0  VLF=1  angleLF=0
      settings: AttributesFormatString=|
      | %<ID>
      | %<Vbase>V
      | %<VLF>pu
      | %<angleLF>deg.
      | %<Name>
  bus5 : powerlib/Measurements/Load Flow Bus  LConnTagsString=a  ID=bus5  Vbase=220000  Vref=1  Vangle=0  VLF=1  angleLF=0
      settings: AttributesFormatString=|
      | %<ID>
      | %<Vbase>V
      | %<VLF>pu
      | %<angleLF>deg.
      | %<Name>
  bus6 : powerlib/Measurements/Load Flow Bus  LConnTagsString=a  ID=bus6  Vbase=220000  Vref=1  Vangle=0  VLF=1  angleLF=0
      settings: AttributesFormatString=|
      | %<ID>
      | %<Vbase>V
      | %<VLF>pu
      | %<angleLF>deg.
      | %<Name>
  bus7 : powerlib/Measurements/Load Flow Bus  LConnTagsString=a  ID=bus7  Vbase=220000  Vref=1  Vangle=0  VLF=1  angleLF=0
      settings: AttributesFormatString=|
      | %<ID>
      | %<Vbase>V
      | %<VLF>pu
      | %<angleLF>deg.
      | %<Name>
  bus8 : powerlib/Measurements/Load Flow Bus  LConnTagsString=a  ID=bus8  Vbase=220000  Vref=1  Vangle=0  VLF=1  angleLF=0
      settings: AttributesFormatString=|
      | %<ID>
      | %<Vbase>V
      | %<VLF>pu
      | %<angleLF>deg.
      | %<Name>
  bus9 : powerlib/Measurements/Load Flow Bus  LConnTagsString=a  ID=bus9  Vbase=220000  Vref=1  Vangle=0  VLF=1  angleLF=0
      settings: AttributesFormatString=|
      | %<ID>
      | %<Vbase>V
      | %<VLF>pu
      | %<angleLF>deg.
      | %<Name>
  powergui : powerlib/powergui  Priority=1  SimulationMode=Continuous  SolverType=Tustin  SampleTime=50e-6  frequency=60  SPID=off  DisableSnubberDevices=off  DisableRonSwitches=off  DisableVfSwitches=off  SwTol=0  Interpol=off  DisplayEquations=off  Ts=0  methode=off  frequencyindice=60  Pbase=100e6  ErrMax=1e-4  Iterations=50  UnitsV=kV  UnitsW=MW  FunctionMessages=off  echomessages=off  HookPort=off  EnableUseOfTLC=off  x0status=blocks  RestoreLinks=warning  ResistiveCurrentMeasurement=off  Frange=[0:2:500]  Ylog=off  Xlog=on  ShowGrid=off  save=off  variable=ZData  structure=0  ZoomFFT=off  StartTime=0.0  cycles=1  DisplayStyle=1  fundamental=60  FreqAxis=off  MaxFrequency=1000  frequencyindicesteady=1  RmsSteady=1  display=off
  connections:
  _CN_307638314_110000_CN_306295536_110000/LConn1 -- T_307638314__/RConn1 -- L_307638314/LConn1
  _CN_307638314_110000_CN_306295536_110000/LConn2 -- T_307638314__/RConn2 -- L_307638314/LConn2
  _CN_307638314_110000_CN_306295536_110000/LConn3 -- T_307638314__/RConn3 -- L_307638314/LConn3 -- bus1/LConn1
  _CN_307638314_110000_CN_306295536_110000/RConn1 -- T_306295536_500000_Trạm_500KV_Nhà_Bè/RConn4 -- L_306295536/LConn1
  _CN_307638314_110000_CN_306295536_110000/RConn2 -- T_306295536_500000_Trạm_500KV_Nhà_Bè/RConn5 -- L_306295536/LConn2
  _CN_307638314_110000_CN_306295536_110000/RConn3 -- T_306295536_500000_Trạm_500KV_Nhà_Bè/RConn6 -- L_306295536/LConn3 -- bus2/LConn1
  T_317106134__/LConn1 -- _CN_317106134_110000_CN_317106135_110000/LConn1
  T_317106134__/LConn2 -- _CN_317106134_110000_CN_317106135_110000/LConn2
  _CN_317106134_110000_CN_317106135_110000/LConn3 -- T_317106134__/LConn3 -- bus3/LConn1
  T_317106135__/LConn1 -- _CN_317106134_110000_CN_317106135_110000/RConn1
  T_317106135__/LConn2 -- _CN_317106134_110000_CN_317106135_110000/RConn2
  _CN_317106134_110000_CN_317106135_110000/RConn3 -- T_317106135__/LConn3 -- bus4/LConn1
  T_308292630__/LConn1 -- _CN_308292630_220000_CN_308292616_220000/LConn1
  T_308292630__/LConn2 -- _CN_308292630_220000_CN_308292616_220000/LConn2
  _CN_308292630_220000_CN_308292616_220000/LConn3 -- T_308292630__/LConn3 -- bus5/LConn1
  G_308292616_/RConn1 -- _CN_308292630_220000_CN_308292616_220000/RConn1
  G_308292616_/RConn2 -- _CN_308292630_220000_CN_308292616_220000/RConn2
  _CN_308292630_220000_CN_308292616_220000/RConn3 -- G_308292616_/RConn3 -- bus6/LConn1
  _CN_306259035_220000_CN_306440155_220000/LConn1 -- T_306259035__/LConn1 -- _CN_306259035_220000_CN_318268202_220000/LConn1 -- _CN_306259035_220000_CN_306259034_220000/LConn1
  _CN_306259035_220000_CN_306440155_220000/LConn2 -- T_306259035__/LConn2 -- _CN_306259035_220000_CN_318268202_220000/LConn2 -- _CN_306259035_220000_CN_306259034_220000/LConn2
  _CN_306259035_220000_CN_306440155_220000/LConn3 -- T_306259035__/LConn3 -- _CN_306259035_220000_CN_318268202_220000/LConn3 -- _CN_306259035_220000_CN_306259034_220000/LConn3 -- bus7/LConn1
  T_306440155__/LConn1 -- _CN_306259035_220000_CN_306440155_220000/RConn1
  T_306440155__/LConn2 -- _CN_306259035_220000_CN_306440155_220000/RConn2
  _CN_306259035_220000_CN_306440155_220000/RConn3 -- T_306440155__/LConn3 -- bus8/LConn1
  T_318268202__/LConn1 -- _CN_306259035_220000_CN_318268202_220000/RConn1
  T_318268202__/LConn2 -- _CN_306259035_220000_CN_318268202_220000/RConn2
  _CN_306259035_220000_CN_318268202_220000/RConn3 -- T_318268202__/LConn3 -- bus9/LConn1
  _CN_306259035_220000_CN_306259034_220000/RConn1 -- T_306259034__/LConn1 -- _CN_306295540_220000_CN_306259034_220000/LConn1
  _CN_306259035_220000_CN_306259034_220000/RConn2 -- T_306259034__/LConn2 -- _CN_306295540_220000_CN_306259034_220000/LConn2
  _CN_306259035_220000_CN_306259034_220000/RConn3 -- T_306259034__/LConn3 -- _CN_306295540_220000_CN_306259034_220000/LConn3 -- bus10/LConn1
  T_307638314__/LConn1 -- _CN_307638314_220000_CN_306295536_220000/LConn1
  T_307638314__/LConn2 -- _CN_307638314_220000_CN_306295536_220000/LConn2
  _CN_307638314_220000_CN_306295536_220000/LConn3 -- T_307638314__/LConn3 -- bus11/LConn1
  _CN_307638314_220000_CN_306295536_220000/RConn1 -- T_306295536_500000_Trạm_500KV_Nhà_Bè/RConn1 -- _CN_306295540_220000_CN_306295536_220000/LConn1
  _CN_307638314_220000_CN_306295536_220000/RConn2 -- T_306295536_500000_Trạm_500KV_Nhà_Bè/RConn2 -- _CN_306295540_220000_CN_306295536_220000/LConn2
  _CN_307638314_220000_CN_306295536_220000/RConn3 -- T_306295536_500000_Trạm_500KV_Nhà_Bè/RConn3 -- _CN_306295540_220000_CN_306295536_220000/LConn3 -- bus12/LConn1
  T_251794098__/LConn1 -- _CN_251794098_220000_CN_251790836_220000/LConn1
  T_251794098__/LConn2 -- _CN_251794098_220000_CN_251790836_220000/LConn2
  _CN_251794098_220000_CN_251790836_220000/LConn3 -- T_251794098__/LConn3 -- bus13/LConn1
  T_251790836__/LConn1 -- _CN_251794098_220000_CN_251790836_220000/RConn1
  T_251790836__/LConn2 -- _CN_251794098_220000_CN_251790836_220000/RConn2
  _CN_251794098_220000_CN_251790836_220000/RConn3 -- T_251790836__/LConn3 -- bus14/LConn1
  _CN_306295540_220000_CN_306295536_220000/RConn1 -- T_306295540__/LConn1 -- _CN_306295540_220000_CN_277519190_220000/LConn1 -- _CN_306295540_220000_CN_306259034_220000/RConn1 -- _CN_306295540_220000_CN_400202736_220000/LConn1
  _CN_306295540_220000_CN_306295536_220000/RConn2 -- T_306295540__/LConn2 -- _CN_306295540_220000_CN_277519190_220000/LConn2 -- _CN_306295540_220000_CN_306259034_220000/RConn2 -- _CN_306295540_220000_CN_400202736_220000/LConn2
  _CN_306295540_220000_CN_306295536_220000/RConn3 -- T_306295540__/LConn3 -- _CN_306295540_220000_CN_277519190_220000/LConn3 -- _CN_306295540_220000_CN_306259034_220000/RConn3 -- _CN_306295540_220000_CN_400202736_220000/LConn3 -- bus15/LConn1
  _CN_306295540_220000_CN_277519190_220000/RConn1 -- T_277519190__/LConn1 -- _CN_277519190_220000_CN_315766015_220000/LConn1
  _CN_306295540_220000_CN_277519190_220000/RConn2 -- T_277519190__/LConn2 -- _CN_277519190_220000_CN_315766015_220000/LConn2
  _CN_306295540_220000_CN_277519190_220000/RConn3 -- T_277519190__/LConn3 -- _CN_277519190_220000_CN_315766015_220000/LConn3 -- bus16/LConn1
  G_400202736_/RConn1 -- _CN_306295540_220000_CN_400202736_220000/RConn1
  G_400202736_/RConn2 -- _CN_306295540_220000_CN_400202736_220000/RConn2
  _CN_306295540_220000_CN_400202736_220000/RConn3 -- G_400202736_/RConn3 -- bus17/LConn1
  T_400413519__/LConn1 -- _CN_400413519_220000_CN_400413521_220000/LConn1
  T_400413519__/LConn2 -- _CN_400413519_220000_CN_400413521_220000/LConn2
  _CN_400413519_220000_CN_400413521_220000/LConn3 -- T_400413519__/LConn3 -- bus18/LConn1
  T_400413521__/LConn1 -- _CN_400413519_220000_CN_400413521_220000/RConn1
  T_400413521__/LConn2 -- _CN_400413519_220000_CN_400413521_220000/RConn2
  _CN_400413519_220000_CN_400413521_220000/RConn3 -- T_400413521__/LConn3 -- bus19/LConn1
  T_315766015__/LConn1 -- _CN_277519190_220000_CN_315766015_220000/RConn1
  T_315766015__/LConn2 -- _CN_277519190_220000_CN_315766015_220000/RConn2
  _CN_277519190_220000_CN_315766015_220000/RConn3 -- T_315766015__/LConn3 -- bus20/LConn1
  _CN_401334056_500000_CN_401447890_500000/LConn1 -- T_401334056__/LConn1 -- _CN_401334056_500000_CN_401274166_500000/LConn1
  _CN_401334056_500000_CN_401447890_500000/LConn2 -- T_401334056__/LConn2 -- _CN_401334056_500000_CN_401274166_500000/LConn2
  _CN_401334056_500000_CN_401447890_500000/LConn3 -- T_401334056__/LConn3 -- _CN_401334056_500000_CN_401274166_500000/LConn3 -- bus21/LConn1
  T_401447890__/LConn1 -- _CN_401334056_500000_CN_401447890_500000/RConn1
  T_401447890__/LConn2 -- _CN_401334056_500000_CN_401447890_500000/RConn2
  _CN_401334056_500000_CN_401447890_500000/RConn3 -- T_401447890__/LConn3 -- bus22/LConn1
  T_401274166__/LConn1 -- _CN_401334056_500000_CN_401274166_500000/RConn1
  T_401274166__/LConn2 -- _CN_401334056_500000_CN_401274166_500000/RConn2
  _CN_401334056_500000_CN_401274166_500000/RConn3 -- T_401274166__/LConn3 -- bus23/LConn1
  _CN_306295536_500000_CN_315553115_500000/LConn1 -- T_306295536_500000_Trạm_500KV_Nhà_Bè/LConn1 -- _CN_306295536_500000_CN_272740093_500000/LConn1
  _CN_306295536_500000_CN_315553115_500000/LConn2 -- T_306295536_500000_Trạm_500KV_Nhà_Bè/LConn2 -- _CN_306295536_500000_CN_272740093_500000/LConn2
  _CN_306295536_500000_CN_315553115_500000/LConn3 -- T_306295536_500000_Trạm_500KV_Nhà_Bè/LConn3 -- _CN_306295536_500000_CN_272740093_500000/LConn3 -- bus24/LConn1
  _CN_306295536_500000_CN_315553115_500000/RConn1 -- T_315553115__Phú_Lâm/LConn1 -- _CN_306440153_500000_CN_315553115_500000/LConn1
  _CN_306295536_500000_CN_315553115_500000/RConn2 -- T_315553115__Phú_Lâm/LConn2 -- _CN_306440153_500000_CN_315553115_500000/LConn2
  _CN_306295536_500000_CN_315553115_500000/RConn3 -- T_315553115__Phú_Lâm/LConn3 -- _CN_306440153_500000_CN_315553115_500000/LConn3 -- bus25/LConn1
  T_272740093_500000_Trạm_500KV_Phú_Mỹ/LConn1 -- _CN_306295536_500000_CN_272740093_500000/RConn1
  T_272740093_500000_Trạm_500KV_Phú_Mỹ/LConn2 -- _CN_306295536_500000_CN_272740093_500000/RConn2
  _CN_306295536_500000_CN_272740093_500000/RConn3 -- T_272740093_500000_Trạm_500KV_Phú_Mỹ/LConn3 -- bus26/LConn1
  T_306440153__/LConn1 -- _CN_306440153_500000_CN_315553115_500000/RConn1
  T_306440153__/LConn2 -- _CN_306440153_500000_CN_315553115_500000/RConn2
  _CN_306440153_500000_CN_315553115_500000/RConn3 -- T_306440153__/LConn3 -- bus27/LConn1
  T_317106134__/RConn1 -- L_317106134/LConn1
  T_317106134__/RConn2 -- L_317106134/LConn2
  L_317106134/LConn3 -- T_317106134__/RConn3 -- bus28/LConn1
  T_317106135__/RConn1 -- L_317106135/LConn1
  T_317106135__/RConn2 -- L_317106135/LConn2
  L_317106135/LConn3 -- T_317106135__/RConn3 -- bus29/LConn1
  T_308292630__/RConn1 -- L_308292630/LConn1
  T_308292630__/RConn2 -- L_308292630/LConn2
  L_308292630/LConn3 -- T_308292630__/RConn3 -- bus30/LConn1
  T_306259035__/RConn1 -- L_306259035/LConn1
  T_306259035__/RConn2 -- L_306259035/LConn2
  L_306259035/LConn3 -- T_306259035__/RConn3 -- bus31/LConn1
  T_306440155__/RConn1 -- L_306440155/LConn1
  T_306440155__/RConn2 -- L_306440155/LConn2
  L_306440155/LConn3 -- T_306440155__/RConn3 -- bus32/LConn1
  T_318268202__/RConn1 -- L_318268202/LConn1
  T_318268202__/RConn2 -- L_318268202/LConn2
  L_318268202/LConn3 -- T_318268202__/RConn3 -- bus33/LConn1
  T_306259034__/RConn1 -- L_306259034/LConn1
  T_306259034__/RConn2 -- L_306259034/LConn2
  L_306259034/LConn3 -- T_306259034__/RConn3 -- bus34/LConn1
  T_251794098__/RConn1 -- L_251794098/LConn1
  T_251794098__/RConn2 -- L_251794098/LConn2
  L_251794098/LConn3 -- T_251794098__/RConn3 -- bus35/LConn1
  T_251790836__/RConn1 -- L_251790836/LConn1
  T_251790836__/RConn2 -- L_251790836/LConn2
  L_251790836/LConn3 -- T_251790836__/RConn3 -- bus36/LConn1
  T_306295540__/RConn1 -- L_306295540/LConn1
  T_306295540__/RConn2 -- L_306295540/LConn2
  L_306295540/LConn3 -- T_306295540__/RConn3 -- bus37/LConn1
  T_277519190__/RConn1 -- L_277519190/LConn1
  T_277519190__/RConn2 -- L_277519190/LConn2
  L_277519190/LConn3 -- T_277519190__/RConn3 -- bus38/LConn1
  T_400413519__/RConn1 -- L_400413519/LConn1
  T_400413519__/RConn2 -- L_400413519/LConn2
  L_400413519/LConn3 -- T_400413519__/RConn3 -- bus39/LConn1
  T_400413521__/RConn1 -- L_400413521/LConn1
  T_400413521__/RConn2 -- L_400413521/LConn2
  L_400413521/LConn3 -- T_400413521__/RConn3 -- bus40/LConn1
  T_315766015__/RConn1 -- L_315766015/LConn1
  T_315766015__/RConn2 -- L_315766015/LConn2
  L_315766015/LConn3 -- T_315766015__/RConn3 -- bus41/LConn1
  T_401334056__/RConn1 -- L_401334056/LConn1
  T_401334056__/RConn2 -- L_401334056/LConn2
  L_401334056/LConn3 -- T_401334056__/RConn3 -- bus42/LConn1
  T_401447890__/RConn1 -- L_401447890/LConn1
  T_401447890__/RConn2 -- L_401447890/LConn2
  L_401447890/LConn3 -- T_401447890__/RConn3 -- bus43/LConn1
  T_401274166__/RConn1 -- L_401274166/LConn1
  T_401274166__/RConn2 -- L_401274166/LConn2
  L_401274166/LConn3 -- T_401274166__/RConn3 -- bus44/LConn1
  T_315553115__Phú_Lâm/RConn1 -- L_315553115/LConn1
  T_315553115__Phú_Lâm/RConn2 -- L_315553115/LConn2
  L_315553115/LConn3 -- T_315553115__Phú_Lâm/RConn3 -- bus45/LConn1
  T_272740093_500000_Trạm_500KV_Phú_Mỹ/RConn1 -- L_272740093/LConn1
  T_272740093_500000_Trạm_500KV_Phú_Mỹ/RConn2 -- L_272740093/LConn2
  L_272740093/LConn3 -- T_272740093_500000_Trạm_500KV_Phú_Mỹ/RConn3 -- bus46/LConn1
  T_306440153__/RConn1 -- L_306440153/LConn1
  T_306440153__/RConn2 -- L_306440153/LConn2
  L_306440153/LConn3 -- T_306440153__/RConn3 -- bus47/LConn1
